simulink model "ServoDriver"  (Simulink 7.0)
settings: Solver=ode45  StartTime=0.0  StopTime=10.0  RelTol=1e-3
settings Model: Creator=volgy  LastModifiedBy=volgy

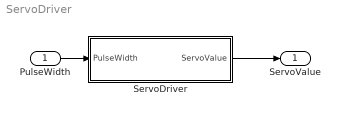
== system ServoDriver ==
  PulseWidth : Inport  OutDataType=sfix(16)  OutScaling=2^0
  ServoDriver : Subsystem
  ServoValue : Outport  OutDataType=sfix(16)  OutScaling=2^0
  wires:
  PulseWidth/1 -> ServoDriver/1(PulseWidth)
  ServoDriver/1(ServoValue) -> ServoValue/1

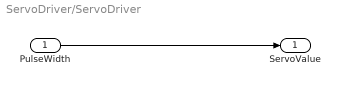
== system ServoDriver/ServoDriver ==
  PulseWidth : Inport  OutDataType=sfix(16)  OutScaling=2^0
  ServoValue : Outport  OutDataType=sfix(16)  OutScaling=2^0
  wires:
  PulseWidth/1 -> ServoValue/1
